simulink model "BaseEngineController_LS"  (Simulink 7.7)
settings: Solver=FixedStepDiscrete  StartTime=0.0  StopTime=10.0  RelTol=1e-3
PreLoadFcn:
  | try, eval([bdroot '_setup']); catch, eval('model_setup', ''); end
InitFcn:
  | try, eval([bdroot '_setup']); catch, eval('model_setup', ''); end
undefined symbols (not defined in the file): ECU555, High, motohawk_build_version, motohawk_trunc_name, motohawk_vardec_config_group, motohawk_vardec_path, True
libraries: MotoHawk_lib x1418, motohawk_control_primitives_lib x183, motohawk_engine_lib x32, simulink x21, motohawk_annotations_lib x9, AutoDoc_lib x8, simulink_extras x4, motohawk_ccp_examples_lib x1, motohawk_control_primitives_motoshare_lib x1
(part 8 of 27)

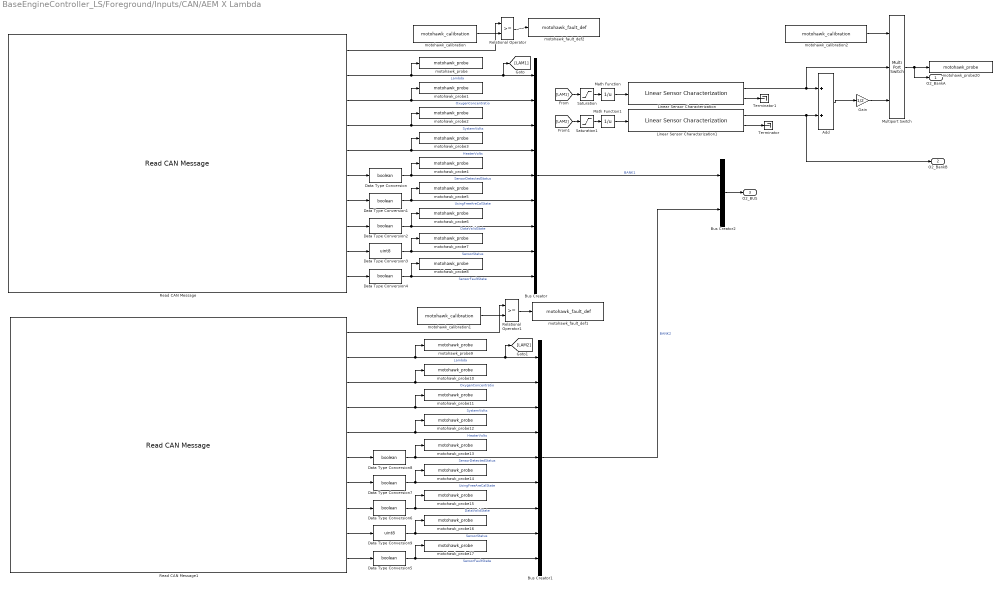
== system BaseEngineController_LS/Foreground/Inputs/CAN/AEM X Lambda ==
  Add : Sum
  Bus Creator : BusCreator  Inputs=9
  Bus Creator1 : BusCreator  Inputs=9
  Bus Creator2 : BusCreator  Inputs=2
  Data Type Conversion{,1..2,4..8} (8 alike) : DataTypeConversion  OutDataTypeStr=boolean
  Data Type Conversion3 : DataTypeConversion  OutDataTypeStr=uint8
  Data Type Conversion9 : DataTypeConversion  OutDataTypeStr=uint8
  Gain : Gain  Gain=1/2
  Linear Sensor Characterization : motohawk_engine_lib/Linear Sensor Characterization  SystemSampleTime=-1  nam='Bank1_EquivRatio'  prefix='Bank1_EquivRatio'  units='EquivRatio'  inputunits='EquivRatio'  parent_group=motohawk_vardec_path(gcb)  samp_time=-1
  Linear Sensor Characterization1 : motohawk_engine_lib/Linear Sensor Characterization  SystemSampleTime=-1  nam='Bank2_EquivRatio'  prefix='Bank2_EquivRatio'  units='EquivRatio'  inputunits='EquivRatio'  parent_group=motohawk_vardec_path(gcb)  samp_time=-1
  Math Function : Math  Operator=reciprocal  SaturateOnIntegerOverflow=on
  Math Function1 : Math  Operator=reciprocal  SaturateOnIntegerOverflow=on
  Multiport Switch : MultiPortSwitch  DataPortOrder=Zero-based contiguous  Inputs=2  zeroidx=on
  Read CAN Message : MotoHawk_lib/CAN Blocks/Read CAN Message  nam='CAN_1'  bus=-2  msg=CANRx_AEM_UEGO_1  queue=1  slot=''  valid=off  stale=on  labelwires=off
  Read CAN Message1 : MotoHawk_lib/CAN Blocks/Read CAN Message  nam='CAN_1'  bus=-2  msg=CANRx_AEM_UEGO_2  queue=1  slot=''  valid=off  stale=on  labelwires=off
  Relational Operator : RelationalOperator  OutDataTypeStr=boolean
  Relational Operator1 : RelationalOperator  OutDataTypeStr=boolean
  Saturation : Saturate  UpperLimit=inf  LowerLimit=.1
  Saturation1 : Saturate  UpperLimit=inf  LowerLimit=.1
  Terminator : Terminator
  Terminator1 : Terminator
  motohawk_calibration : MotoHawk_lib/Calibration & Probing Blocks/motohawk_calibration  nam='Lambda_1_Timeout'  val=100  storage=Calibration  show_more=on  name_source=Use Parameter  data_type=uint16  read_level=1  write_level=1  ovr_cals=on  view_as=Number  enum_struct={'Disabled', 'Enabled'}  vector_style=Wide Row  use_help_units=on  help=''  units='ms'  use_header_enum=off  row_header_enum={}  col_header_enum={}  use_min_max=off  min_val=-inf  max_val=inf  use_precision=off  precision=''  gain=1  offset=0  exp=1  use_mototune_group=off  mototune_group=motohawk_vardec_path(gcb)
  motohawk_calibration1 : MotoHawk_lib/Calibration & Probing Blocks/motohawk_calibration  nam='Lambda_2_Timeout'  val=100  storage=Calibration  show_more=on  name_source=Use Parameter  data_type=uint16  read_level=1  write_level=1  ovr_cals=on  view_as=Number  enum_struct={'Disabled', 'Enabled'}  vector_style=Wide Row  use_help_units=on  help=''  units='ms'  use_header_enum=off  row_header_enum={}  col_header_enum={}  use_min_max=off  min_val=-inf  max_val=inf  use_precision=off  precision=''  gain=1  offset=0  exp=1  use_mototune_group=off  mototune_group=motohawk_vardec_path(gcb)
  motohawk_calibration2 : MotoHawk_lib/Calibration & Probing Blocks/motohawk_calibration  nam='BankB_Avg_Enable'  val=1  storage=Calibration  show_more=on  name_source=Use Parameter  data_type=boolean  read_level=1  write_level=1  ovr_cals=on  view_as=Enumeration  enum_struct={'Disabled', 'Enabled'}  vector_style=Wide Row  use_help_units=off  help=''  units=''  use_header_enum=off  row_header_enum={}  col_header_enum={}  use_min_max=off  min_val=-inf  max_val=inf  use_precision=off  precision=''  gain=1  offset=0  exp=1  use_mototune_group=off  mototune_group=motohawk_vardec_path(gcb)
  motohawk_fault_def1 : MotoHawk_lib/Fault Management Blocks/motohawk_fault_def  nam='Lambda_2_Timeout'  mode=Enabled  id=[]  x=1  y=2  input_suspected=on  indeterminate=off  increment_xy=on  downsample_count=1  ovr_cals=on  ovr_actions=on  show_actions=on  action1_name=''  action1_cond=(None)  action2_name=''  action2_cond=(None)  action3_name=''  action3_cond=(None)  action4_name=''  action4_cond=(None)
  motohawk_fault_def2 : MotoHawk_lib/Fault Management Blocks/motohawk_fault_def  nam='Lambda_1_Timeout'  mode=Enabled  id=[]  x=1  y=2  input_suspected=on  indeterminate=off  increment_xy=on  downsample_count=1  ovr_cals=on  ovr_actions=on  show_actions=on  action1_name=''  action1_cond=(None)  action2_name=''  action2_cond=(None)  action3_name=''  action3_cond=(None)  action4_name=''  action4_cond=(None)
  motohawk_probe : MotoHawk_lib/Calibration & Probing Blocks/motohawk_probe  nam='Bank1_Lambda_Prb'  show_more=off  name_source=Use Parameter  read_level=1  view_as=Number  enum_struct={'Disabled', 'Enabled'}  vector_style=Wide Row  use_help_units=off  help=''  units=''  use_header_enum=off  row_header_enum={}  col_header_enum={}  use_precision=off  precision=''  gain=1  offset=0  exp=1  use_mototune_group=off  mototune_group=motohawk_vardec_path(gcb)
  motohawk_probe1 : MotoHawk_lib/Calibration & Probing Blocks/motohawk_probe  nam='Bank1_OxygenConcentration_Prb'  show_more=off  name_source=Use Parameter  read_level=1  view_as=Number  enum_struct={'Disabled', 'Enabled'}  vector_style=Wide Row  use_help_units=off  help=''  units=''  use_header_enum=off  row_header_enum={}  col_header_enum={}  use_precision=off  precision=''  gain=1  offset=0  exp=1  use_mototune_group=off  mototune_group=motohawk_vardec_path(gcb)
  motohawk_probe10 : MotoHawk_lib/Calibration & Probing Blocks/motohawk_probe  nam='Bank2_OxygenConcentration_Prb'  show_more=off  name_source=Use Parameter  read_level=1  view_as=Number  enum_struct={'Disabled', 'Enabled'}  vector_style=Wide Row  use_help_units=off  help=''  units=''  use_header_enum=off  row_header_enum={}  col_header_enum={}  use_precision=off  precision=''  gain=1  offset=0  exp=1  use_mototune_group=off  mototune_group=motohawk_vardec_path(gcb)
  motohawk_probe11 : MotoHawk_lib/Calibration & Probing Blocks/motohawk_probe  nam='Bank2_SystemVolts_Prb'  show_more=off  name_source=Use Parameter  read_level=1  view_as=Number  enum_struct={'Disabled', 'Enabled'}  vector_style=Wide Row  use_help_units=off  help=''  units=''  use_header_enum=off  row_header_enum={}  col_header_enum={}  use_precision=off  precision=''  gain=1  offset=0  exp=1  use_mototune_group=off  mototune_group=motohawk_vardec_path(gcb)
  motohawk_probe12 : MotoHawk_lib/Calibration & Probing Blocks/motohawk_probe  nam='Bank2_HeaterVolts_Prb'  show_more=off  name_source=Use Parameter  read_level=1  view_as=Number  enum_struct={'Disabled', 'Enabled'}  vector_style=Wide Row  use_help_units=off  help=''  units=''  use_header_enum=off  row_header_enum={}  col_header_enum={}  use_precision=off  precision=''  gain=1  offset=0  exp=1  use_mototune_group=off  mototune_group=motohawk_vardec_path(gcb)
  motohawk_probe13 : MotoHawk_lib/Calibration & Probing Blocks/motohawk_probe  nam='Bank2_SensorDetectedStatus_Prb'  show_more=off  name_source=Use Parameter  read_level=1  view_as=Number  enum_struct={'Disabled', 'Enabled'}  vector_style=Wide Row  use_help_units=off  help=''  units=''  use_header_enum=off  row_header_enum={}  col_header_enum={}  use_precision=off  precision=''  gain=1  offset=0  exp=1  use_mototune_group=off  mototune_group=motohawk_vardec_path(gcb)
  motohawk_probe14 : MotoHawk_lib/Calibration & Probing Blocks/motohawk_probe  nam='Bank2_UsingFreeAreCalState_Prb'  show_more=off  name_source=Use Parameter  read_level=1  view_as=Number  enum_struct={'Disabled', 'Enabled'}  vector_style=Wide Row  use_help_units=off  help=''  units=''  use_header_enum=off  row_header_enum={}  col_header_enum={}  use_precision=off  precision=''  gain=1  offset=0  exp=1  use_mototune_group=off  mototune_group=motohawk_vardec_path(gcb)
  motohawk_probe15 : MotoHawk_lib/Calibration & Probing Blocks/motohawk_probe  nam='Bank2_DataValidState_Prb'  show_more=off  name_source=Use Parameter  read_level=1  view_as=Number  enum_struct={'Disabled', 'Enabled'}  vector_style=Wide Row  use_help_units=off  help=''  units=''  use_header_enum=off  row_header_enum={}  col_header_enum={}  use_precision=off  precision=''  gain=1  offset=0  exp=1  use_mototune_group=off  mototune_group=motohawk_vardec_path(gcb)
  motohawk_probe16 : MotoHawk_lib/Calibration & Probing Blocks/motohawk_probe  nam='Bank2_SensorStatus_Prb'  show_more=on  name_source=Use Parameter  read_level=1  view_as=Enumeration  enum_struct={'Reset', 'WarmingUp', ' Stabilizing', 'ReadingNerstPumpImpedance', 'Equalizing', 'ReadingRcalValue', 'Run', 'Overheat', 'Overcool', 'HeaterShortCircuit', 'HeaterOpenCircuit', 'StartFreeAirCal', 'PerformingFreeAirCal', 'DetectingSensor', 'ReadingJunctionImpedance', 'EvapStartup', 'DeterminingSensorType', 'PreparingToRun','SaveSensor','NeedsNewFreeAirCal','Error'}  vector_style=Wide Row  use_help_units=off  help=''  units=''  use_header_enum=off  row_header_enum={}  col_header_enum={}  use_precision=off  precision=''  gain=1  offset=0  exp=1  use_mototune_group=off  mototune_group=motohawk_vardec_path(gcb)
  motohawk_probe17 : MotoHawk_lib/Calibration & Probing Blocks/motohawk_probe  nam='Bank2_SensorFaultState_Prb'  show_more=off  name_source=Use Parameter  read_level=1  view_as=Number  enum_struct={'Disabled', 'Enabled'}  vector_style=Wide Row  use_help_units=off  help=''  units=''  use_header_enum=off  row_header_enum={}  col_header_enum={}  use_precision=off  precision=''  gain=1  offset=0  exp=1  use_mototune_group=off  mototune_group=motohawk_vardec_path(gcb)
  motohawk_probe2 : MotoHawk_lib/Calibration & Probing Blocks/motohawk_probe  nam='Bank1_SystemVolts_Prb'  show_more=off  name_source=Use Parameter  read_level=1  view_as=Number  enum_struct={'Disabled', 'Enabled'}  vector_style=Wide Row  use_help_units=off  help=''  units=''  use_header_enum=off  row_header_enum={}  col_header_enum={}  use_precision=off  precision=''  gain=1  offset=0  exp=1  use_mototune_group=off  mototune_group=motohawk_vardec_path(gcb)
  motohawk_probe20 : MotoHawk_lib/Calibration & Probing Blocks/motohawk_probe  nam='O2_BankA_EquivRatio_Out'  show_more=off  name_source=Use Parameter  read_level=1  view_as=Number  enum_struct={'Disabled', 'Enabled'}  vector_style=Wide Row  use_help_units=off  help=''  units=''  use_header_enum=off  row_header_enum={}  col_header_enum={}  use_precision=off  precision=''  gain=1  offset=0  exp=1  use_mototune_group=off  mototune_group=motohawk_vardec_path(gcb)
  motohawk_probe3 : MotoHawk_lib/Calibration & Probing Blocks/motohawk_probe  nam='Bank1_HeaterVolts_Prb'  show_more=off  name_source=Use Parameter  read_level=1  view_as=Number  enum_struct={'Disabled', 'Enabled'}  vector_style=Wide Row  use_help_units=off  help=''  units=''  use_header_enum=off  row_header_enum={}  col_header_enum={}  use_precision=off  precision=''  gain=1  offset=0  exp=1  use_mototune_group=off  mototune_group=motohawk_vardec_path(gcb)
  motohawk_probe4 : MotoHawk_lib/Calibration & Probing Blocks/motohawk_probe  nam='Bank1_SensorDetectedStatus_Prb'  show_more=off  name_source=Use Parameter  read_level=1  view_as=Number  enum_struct={'Disabled', 'Enabled'}  vector_style=Wide Row  use_help_units=off  help=''  units=''  use_header_enum=off  row_header_enum={}  col_header_enum={}  use_precision=off  precision=''  gain=1  offset=0  exp=1  use_mototune_group=off  mototune_group=motohawk_vardec_path(gcb)
  motohawk_probe5 : MotoHawk_lib/Calibration & Probing Blocks/motohawk_probe  nam='Bank1_UsingFreeAreCalState_Prb'  show_more=off  name_source=Use Parameter  read_level=1  view_as=Number  enum_struct={'Disabled', 'Enabled'}  vector_style=Wide Row  use_help_units=off  help=''  units=''  use_header_enum=off  row_header_enum={}  col_header_enum={}  use_precision=off  precision=''  gain=1  offset=0  exp=1  use_mototune_group=off  mototune_group=motohawk_vardec_path(gcb)
  motohawk_probe6 : MotoHawk_lib/Calibration & Probing Blocks/motohawk_probe  nam='Bank1_DataValidState_Prb'  show_more=off  name_source=Use Parameter  read_level=1  view_as=Number  enum_struct={'Disabled', 'Enabled'}  vector_style=Wide Row  use_help_units=off  help=''  units=''  use_header_enum=off  row_header_enum={}  col_header_enum={}  use_precision=off  precision=''  gain=1  offset=0  exp=1  use_mototune_group=off  mototune_group=motohawk_vardec_path(gcb)
  motohawk_probe7 : MotoHawk_lib/Calibration & Probing Blocks/motohawk_probe  nam='Bank1_SensorStatus_Prb'  show_more=on  name_source=Use Parameter  read_level=1  view_as=Enumeration  enum_struct={'Reset', 'WarmingUp', ' Stabilizing', 'ReadingNerstPumpImpedance', 'Equalizing', 'ReadingRcalValue', 'Run', 'Overheat', 'Overcool', 'HeaterShortCircuit', 'HeaterOpenCircuit', 'StartFreeAirCal', 'PerformingFreeAirCal', 'DetectingSensor', 'ReadingJunctionImpedance', 'EvapStartup', 'DeterminingSensorType', 'PreparingToRun','SaveSensor','NeedsNewFreeAirCal','Error'}  vector_style=Wide Row  use_help_units=off  help=''  units=''  use_header_enum=off  row_header_enum={}  col_header_enum={}  use_precision=off  precision=''  gain=1  offset=0  exp=1  use_mototune_group=off  mototune_group=motohawk_vardec_path(gcb)
  motohawk_probe8 : MotoHawk_lib/Calibration & Probing Blocks/motohawk_probe  nam='Bank1_SensorFaultState_Prb'  show_more=off  name_source=Use Parameter  read_level=1  view_as=Number  enum_struct={'Disabled', 'Enabled'}  vector_style=Wide Row  use_help_units=off  help=''  units=''  use_header_enum=off  row_header_enum={}  col_header_enum={}  use_precision=off  precision=''  gain=1  offset=0  exp=1  use_mototune_group=off  mototune_group=motohawk_vardec_path(gcb)
  motohawk_probe9 : MotoHawk_lib/Calibration & Probing Blocks/motohawk_probe  nam='Bank2_Lambda_Prb'  show_more=off  name_source=Use Parameter  read_level=1  view_as=Number  enum_struct={'Disabled', 'Enabled'}  vector_style=Wide Row  use_help_units=off  help=''  units=''  use_header_enum=off  row_header_enum={}  col_header_enum={}  use_precision=off  precision=''  gain=1  offset=0  exp=1  use_mototune_group=off  mototune_group=motohawk_vardec_path(gcb)
  O2_BankA : Outport
  O2_BankB : Outport  Port=2
  O2_BUS : Outport  Port=3
  wires:
  Read CAN Message/1 -> Relational Operator/1
  motohawk_calibration/1 -> Relational Operator/2
  Relational Operator/1 -> motohawk_fault_def2/1
  Read CAN Message/2 -> motohawk_probe/1, Bus Creator/1, [LAM1]  "Lambda"
  Read CAN Message/3 -> motohawk_probe1/1, Bus Creator/2  "OxygenConcentratio"
  Read CAN Message/4 -> motohawk_probe2/1, Bus Creator/3  "SystemVolts"
  Read CAN Message/5 -> motohawk_probe3/1, Bus Creator/4  "HeaterVolts"
  Read CAN Message/6 -> Data Type Conversion/1
  Read CAN Message/7 -> Data Type Conversion1/1
  Read CAN Message/8 -> Data Type Conversion2/1
  Read CAN Message/9 -> Data Type Conversion3/1
  Read CAN Message/10 -> Data Type Conversion4/1
  Read CAN Message1/1 -> Relational Operator1/1
  motohawk_calibration1/1 -> Relational Operator1/2
  Relational Operator1/1 -> motohawk_fault_def1/1
  Read CAN Message1/2 -> motohawk_probe9/1, Bus Creator1/1, [LAM2]  "Lambda"
  Read CAN Message1/3 -> motohawk_probe10/1, Bus Creator1/2  "OxygenConcentratio"
  Read CAN Message1/4 -> motohawk_probe11/1, Bus Creator1/3  "SystemVolts"
  Read CAN Message1/5 -> motohawk_probe12/1, Bus Creator1/4  "HeaterVolts"
  Read CAN Message1/6 -> Data Type Conversion8/1
  Read CAN Message1/7 -> Data Type Conversion7/1
  Read CAN Message1/8 -> Data Type Conversion6/1
  Read CAN Message1/9 -> Data Type Conversion9/1
  Read CAN Message1/10 -> Data Type Conversion5/1
  Bus Creator/1 -> Bus Creator2/1  "BANK1"
  Bus Creator1/1 -> Bus Creator2/2  "BANK2"
  Bus Creator2/1 -> O2_BUS/1
  [LAM1] -> Saturation/1
  [LAM2] -> Saturation1/1
  Math Function/1 -> Linear Sensor Characterization/1
  Math Function1/1 -> Linear Sensor Characterization1/1
  Linear Sensor Characterization1/2 -> Terminator/1
  Linear Sensor Characterization/2 -> Terminator1/1
  Linear Sensor Characterization/1 -> Add/1, Multiport Switch/2
  Add/1 -> Gain/1
  motohawk_calibration2/1 -> Multiport Switch/1
  Saturation/1 -> Math Function/1
  Saturation1/1 -> Math Function1/1
  Linear Sensor Characterization1/1 -> Add/2, O2_BankB/1
  Multiport Switch/1 -> O2_BankA/1, motohawk_probe20/1
  Gain/1 -> Multiport Switch/3
  Data Type Conversion/1 -> motohawk_probe4/1, Bus Creator/5  "SensorDetectedStatus"
  Data Type Conversion1/1 -> motohawk_probe5/1, Bus Creator/6  "UsingFreeAreCalState"
  Data Type Conversion2/1 -> motohawk_probe6/1, Bus Creator/7  "DataValidState"
  Data Type Conversion3/1 -> motohawk_probe7/1, Bus Creator/8  "SensorStatus"
  Data Type Conversion4/1 -> motohawk_probe8/1, Bus Creator/9  "SensorFaultState"
  Data Type Conversion5/1 -> motohawk_probe17/1, Bus Creator1/9  "SensorFaultState"
  Data Type Conversion6/1 -> motohawk_probe15/1, Bus Creator1/7  "DataValidState"
  Data Type Conversion7/1 -> motohawk_probe14/1, Bus Creator1/6  "UsingFreeAreCalState"
  Data Type Conversion8/1 -> motohawk_probe13/1, Bus Creator1/5  "SensorDetectedStatus"
  Data Type Conversion9/1 -> motohawk_probe16/1, Bus Creator1/8  "SensorStatus"

== system BaseEngineController_LS/Foreground/Inputs/Digital/Scramble  ==
  ADC : Inport
  0 = No Inversion 1 = Inversion : MotoHawk_lib/Calibration & Probing Blocks/motohawk_calibration  nam=[prefix 'Polarity']  val=boolean(polarity-1)  storage=Calibration  show_more=on  name_source=Use Parameter  data_type=Inherit from 'Default Value'  read_level=1  write_level=1  ovr_cals=on  view_as=Number  enum_struct={'Disabled', 'Enabled'}  vector_style=Wide Row  use_help_units=on  help="'0 = High True    1 = Low True'"  units='bool'  use_header_enum=off  row_header_enum={}  col_header_enum={}  use_min_max=off  min_val=-inf  max_val=inf  use_precision=off  precision=''  gain=1  offset=0  exp=1  use_mototune_group=on  mototune_group=[group ' | ' nam ' Config']
  Button Delay 1 : Subsystem
  Data Type Conversion : DataTypeConversion  SaturateOnIntegerOverflow=on  RndMeth=Zero
  Logical Operator : Logic  Operator=XOR
  Override in Engineering Units : MotoHawk_lib/Calibration & Probing Blocks/motohawk_override_abs  SystemSampleTime=-1  parent_name=nam  parent_val=0  show_more=on  name_source=Use Parameter  parent_read_level=1  parent_override_level=1  view_as=Number  enum_struct={'Disabled', 'Enabled'}  use_help_units=on  parent_help='Override actuator, in engineering units'  parent_units='Boolean'  use_min_max=off  parent_min=-inf  parent_max=inf  use_precision=off  parent_precision=''  parent_gain=1  parent_offset=0  parent_exp=1  use_mototune_group=on  parent_group=group
  Relational Operator : RelationalOperator  Operator=>
  SwitchPoint : MotoHawk_lib/Calibration & Probing Blocks/motohawk_calibration  nam=[prefix 'SwitchPt']  val=switchpoint  storage=Calibration  show_more=on  name_source=Use Parameter  data_type=Inherit from 'Default Value'  read_level=1  write_level=1  ovr_cals=on  view_as=Number  enum_struct={'Disabled', 'Enabled'}  vector_style=Wide Row  use_help_units=on  help='Defines switch point in ADC units boolean conversion'  units='ADC'  use_header_enum=off  row_header_enum={}  col_header_enum={}  use_min_max=off  min_val=-inf  max_val=inf  use_precision=off  precision=''  gain=1  offset=0  exp=1  use_mototune_group=on  mototune_group=[group ' | ' nam ' Config']
  motohawk_calibration7 : MotoHawk_lib/Calibration & Probing Blocks/motohawk_calibration  nam='ScrambleDebounceDelay'  val=0.08  storage=Calibration  show_more=on  name_source=Use Parameter  data_type=Inherit from 'Default Value'  read_level=1  write_level=1  ovr_cals=on  view_as=Number  enum_struct={'Disabled', 'Enabled'}  vector_style=Wide Row  use_help_units=on  help='Cruise control debounce time'  units='S'  use_header_enum=off  row_header_enum={}  col_header_enum={}  use_min_max=off  min_val=-inf  max_val=inf  use_precision=off  precision=''  gain=1  offset=0  exp=1  use_mototune_group=off  mototune_group=motohawk_vardec_path(gcb)
  motohawk_probe : MotoHawk_lib/Calibration & Probing Blocks/motohawk_probe  nam=nam  show_more=on  name_source=Use Parameter  read_level=1  view_as=Number  enum_struct={'Disabled', 'Enabled'}  vector_style=Wide Row  use_help_units=on  help='Display output in engineering units'  units='Boolean'  use_header_enum=off  row_header_enum={}  col_header_enum={}  use_precision=off  precision=''  gain=1  offset=0  exp=1  use_mototune_group=on  mototune_group=group
  motohawk_probe1 : MotoHawk_lib/Calibration & Probing Blocks/motohawk_probe  nam=[nam '_Raw']  show_more=on  name_source=Use Parameter  read_level=1  view_as=Number  enum_struct={'Disabled', 'Enabled'}  vector_style=Wide Row  use_help_units=on  help='Display output in engineering units'  units='ADC'  use_header_enum=off  row_header_enum={}  col_header_enum={}  use_precision=off  precision=''  gain=1  offset=0  exp=1  use_mototune_group=on  mototune_group=group
  DiscOut : Outport
  wires:
  ADC/1 -> Data Type Conversion/1
  0 = No Inversion 1 = Inversion/1 -> Logical Operator/2
  Relational Operator/1 -> Logical Operator/1
  SwitchPoint/1 -> Relational Operator/2
  Override in Engineering Units/1 -> DiscOut/1, motohawk_probe/1
  Data Type Conversion/1 -> Relational Operator/1, motohawk_probe1/1
  motohawk_calibration7/1 -> Button Delay 1/2(Time)
  Logical Operator/1 -> Button Delay 1/1(In1)
  Button Delay 1/1(Out1) -> Override in Engineering Units/1

== system BaseEngineController_LS/Foreground/Inputs/Digital/VSPD_Filt ==
  In1 : Inport
  Abs : Abs
  Abs1 : Abs
  Abs2 : Abs
  Derivitive : motohawk_control_primitives_lib/Derivitive  SystemSampleTime=-1  samp_time=-1
  Logical Operator : Logic  AllPortsSameDT=off  OutDataTypeStr=boolean
  Logical Operator1 : Logic  Operator=OR  AllPortsSameDT=off  OutDataTypeStr=boolean
  Logical Operator2 : Logic  AllPortsSameDT=off  OutDataTypeStr=boolean
  Logical Operator3 : Logic  AllPortsSameDT=off  OutDataTypeStr=boolean
  Logical Operator5 : Logic  Operator=OR  AllPortsSameDT=off  OutDataTypeStr=boolean
  Relational Operator : RelationalOperator  OutDataTypeStr=boolean
  Relational Operator1 : RelationalOperator  Operator=<=  OutDataTypeStr=boolean
  Relational Operator2 : RelationalOperator  OutDataTypeStr=boolean
  Relational Operator3 : RelationalOperator  OutDataTypeStr=boolean
  S-R Flip-Flop : simulink_extras/Flip Flops/S-R Flip-Flop  SystemSampleTime=-1  initial_condition=0
  Sum : Sum  Inputs=+-
  Switch : Switch  Criteria=u2 ~= 0
  Terminator : Terminator
  Time Since Enabled (With Input)1 : motohawk_control_primitives_lib/Time Since Enabled (With Input)1  SystemSampleTime=-1  nam='TimeSinceVSPDReject'  samp_time=-1  init=0  upperlim=16000
  Unit Delay{,1..3} (4 alike) : UnitDelay  SampleTime=-1
  motohawk_calibration1 : MotoHawk_lib/Calibration & Probing Blocks/motohawk_calibration  nam='VSPD_RateReject_Enable'  val=1  storage=Calibration  show_more=on  name_source=Use Parameter  data_type=boolean  read_level=1  write_level=1  ovr_cals=on  view_as=Enumeration  enum_struct={'Disabled', 'Enabled'}  vector_style=Wide Row  use_help_units=on  help='Enable for if VSPD changes by more than this per/second ignore it'  units='enum'  use_header_enum=off  row_header_enum={}  col_header_enum={}  use_min_max=off  min_val=-inf  max_val=inf  use_precision=off  precision=''  gain=1  offset=0  exp=1  use_mototune_group=off  mototune_group=motohawk_vardec_path(gcb)
  motohawk_calibration2 : MotoHawk_lib/Calibration & Probing Blocks/motohawk_calibration  nam='VSPD_RateReject'  val=300  storage=Calibration  show_more=on  name_source=Use Parameter  data_type=Inherit via back propagation  read_level=1  write_level=1  ovr_cals=on  view_as=Number  enum_struct={'Disabled', 'Enabled'}  vector_style=Wide Row  use_help_units=on  help='If VSPD changes by more than this per/second ignore it'  units='mph/s'  use_header_enum=off  row_header_enum={}  col_header_enum={}  use_min_max=off  min_val=-inf  max_val=inf  use_precision=off  precision=''  gain=1  offset=0  exp=1  use_mototune_group=off  mototune_group=motohawk_vardec_path(gcb)
  motohawk_calibration3 : MotoHawk_lib/Calibration & Probing Blocks/motohawk_calibration  nam='VSPD_ZeroSpeed'  val=0.01  storage=Calibration  show_more=on  name_source=Use Parameter  data_type=Inherit from 'Default Value'  read_level=1  write_level=1  ovr_cals=on  view_as=Number  enum_struct={'Disabled', 'Enabled'}  vector_style=Wide Row  use_help_units=on  help='What VSPD filter considers zero speed'  units='mph'  use_header_enum=off  row_header_enum={}  col_header_enum={}  use_min_max=off  min_val=-inf  max_val=inf  use_precision=off  precision=''  gain=1  offset=0  exp=1  use_mototune_group=off  mototune_group=motohawk_vardec_path(gcb)
  motohawk_calibration4 : MotoHawk_lib/Calibration & Probing Blocks/motohawk_calibration  nam='VPSD_ChangeReject'  val=10  storage=Calibration  show_more=on  name_source=Use Parameter  data_type=Inherit via back propagation  read_level=1  write_level=1  ovr_cals=on  view_as=Number  enum_struct={'Disabled', 'Enabled'}  vector_style=Wide Row  use_help_units=on  help='If VSPD changes by more than this per/second ignore it'  units='mph/s'  use_header_enum=off  row_header_enum={}  col_header_enum={}  use_min_max=off  min_val=-inf  max_val=inf  use_precision=off  precision=''  gain=1  offset=0  exp=1  use_mototune_group=off  mototune_group=motohawk_vardec_path(gcb)
  motohawk_calibration5 : MotoHawk_lib/Calibration & Probing Blocks/motohawk_calibration  nam='VSPD_ChangeReject_Enable'  val=1  storage=Calibration  show_more=on  name_source=Use Parameter  data_type=boolean  read_level=1  write_level=1  ovr_cals=on  view_as=Enumeration  enum_struct={'Disabled', 'Enabled'}  vector_style=Wide Row  use_help_units=on  help='Enable for if VSPD changes by more than this per/second ignore it'  units='enum'  use_header_enum=off  row_header_enum={}  col_header_enum={}  use_min_max=off  min_val=-inf  max_val=inf  use_precision=off  precision=''  gain=1  offset=0  exp=1  use_mototune_group=off  mototune_group=motohawk_vardec_path(gcb)
  motohawk_calibration6 : MotoHawk_lib/Calibration & Probing Blocks/motohawk_calibration  nam='VSPD_RejectHoldTime'  val=1  storage=Calibration  show_more=on  name_source=Use Parameter  data_type=uint8  read_level=1  write_level=1  ovr_cals=on  view_as=Number  enum_struct={'Disabled', 'Enabled'}  vector_style=Wide Row  use_help_units=on  help='TimeToHoldLastValue'  units='sec'  use_header_enum=off  row_header_enum={}  col_header_enum={}  use_min_max=off  min_val=-inf  max_val=inf  use_precision=off  precision=''  gain=1  offset=0  exp=1  use_mototune_group=off  mototune_group=motohawk_vardec_path(gcb)
  motohawk_probe : MotoHawk_lib/Calibration & Probing Blocks/motohawk_probe  nam='VSPD_RateReject_Enabled'  show_more=off  name_source=Use Parameter  read_level=1  view_as=Number  enum_struct={'Disabled', 'Enabled'}  vector_style=Wide Row  use_help_units=off  help=''  units=''  use_header_enum=off  row_header_enum={}  col_header_enum={}  use_precision=off  precision=''  gain=1  offset=0  exp=1  use_mototune_group=off  mototune_group=motohawk_vardec_path(gcb)
  motohawk_probe1 : MotoHawk_lib/Calibration & Probing Blocks/motohawk_probe  nam='VSPD_ChangeReject_Enabled'  show_more=off  name_source=Use Parameter  read_level=1  view_as=Number  enum_struct={'Disabled', 'Enabled'}  vector_style=Wide Row  use_help_units=off  help=''  units=''  use_header_enum=off  row_header_enum={}  col_header_enum={}  use_precision=off  precision=''  gain=1  offset=0  exp=1  use_mototune_group=off  mototune_group=motohawk_vardec_path(gcb)
  motohawk_probe2 : MotoHawk_lib/Calibration & Probing Blocks/motohawk_probe  nam='VSPD_DigFinal'  show_more=off  name_source=Use Parameter  read_level=1  view_as=Number  enum_struct={'Disabled', 'Enabled'}  vector_style=Wide Row  use_help_units=off  help=''  units=''  use_header_enum=off  row_header_enum={}  col_header_enum={}  use_precision=off  precision=''  gain=1  offset=0  exp=1  use_mototune_group=off  mototune_group=motohawk_vardec_path(gcb)
  Out1 : Outport
  wires:
  In1/1 -> Derivitive/1, Sum/1, Abs1/1, Unit Delay1/1, Unit Delay3/1
  Derivitive/1 -> Abs/1
  Abs/1 -> Relational Operator/1
  motohawk_calibration2/1 -> Relational Operator/2
  Switch/1 -> Unit Delay/1, motohawk_probe2/1, Out1/1
  Unit Delay/1 -> Switch/1
  Relational Operator/1 -> Logical Operator/1
  motohawk_calibration1/1 -> Logical Operator/2
  Unit Delay1/1 -> Sum/2
  Abs1/1 -> Relational Operator1/1
  motohawk_calibration3/1 -> Relational Operator1/2
  Sum/1 -> Abs2/1
  motohawk_calibration4/1 -> Relational Operator2/2
  Abs2/1 -> Relational Operator2/1
  Relational Operator2/1 -> Logical Operator2/1
  Relational Operator1/1 -> Logical Operator2/2
  Logical Operator2/1 -> Logical Operator3/1
  motohawk_calibration5/1 -> Logical Operator3/2
  Logical Operator1/1 -> Logical Operator5/2, S-R Flip-Flop/1
  Logical Operator/1 -> Logical Operator1/1, motohawk_probe/1
  Logical Operator3/1 -> Logical Operator1/2, motohawk_probe1/1
  Time Since Enabled (With Input)1/1 -> Relational Operator3/1
  motohawk_calibration6/1 -> Relational Operator3/2
  S-R Flip-Flop/1 -> Logical Operator5/1, Time Since Enabled (With Input)1/1
  Logical Operator5/1 -> Switch/2
  Relational Operator3/1 -> Unit Delay2/1
  Unit Delay2/1 -> S-R Flip-Flop/2
  S-R Flip-Flop/2 -> Terminator/1
  Unit Delay3/1 -> Switch/3

== system BaseEngineController_LS/Foreground/Inputs/EngineSpeed/Encoder Diagnostics ==
  Encoder Fault : Inport
  CamEdges : motohawk_control_primitives_lib/CompareTo  SystemSampleTime=-1  op===  val=4
  CamSync : motohawk_control_primitives_lib/CompareTo  SystemSampleTime=-1  op===  val=5
  CounterThresh : motohawk_control_primitives_lib/CompareTo  SystemSampleTime=-1  op=>  val=100
  CrankEdges : motohawk_control_primitives_lib/CompareTo  SystemSampleTime=-1  op===  val=3
  CrankSync : motohawk_control_primitives_lib/CompareTo  SystemSampleTime=-1  op===  val=1
  Logical Operator{,1..3} (4 alike) : Logic  AllPortsSameDT=off  OutDataTypeStr=boolean
  motohawk_encoder_fault_trigger : MotoHawk_lib/Encoder Blocks/motohawk_encoder_fault_trigger  Tag=Trigger  inherited=on
  motohawk_fault_def : MotoHawk_lib/Fault Management Blocks/motohawk_fault_def  nam='CrankSyncFault'  mode=Enabled  id=[]  x=25  y=50  input_suspected=on  indeterminate=off  increment_xy=on  downsample_count=1  ovr_cals=on  ovr_actions=on  show_actions=off  action1_name=''  action1_cond=(None)  action2_name=''  action2_cond=(None)  action3_name=''  action3_cond=(None)  action4_name=''  action4_cond=(None)
  motohawk_fault_def1 : MotoHawk_lib/Fault Management Blocks/motohawk_fault_def  nam='CrankEdgesFault'  mode=Enabled  id=[]  x=25  y=50  input_suspected=on  indeterminate=off  increment_xy=on  downsample_count=1  ovr_cals=on  ovr_actions=on  show_actions=off  action1_name=''  action1_cond=(None)  action2_name=''  action2_cond=(None)  action3_name=''  action3_cond=(None)  action4_name=''  action4_cond=(None)
  motohawk_fault_def2 : MotoHawk_lib/Fault Management Blocks/motohawk_fault_def  nam='CamEdgesFault'  mode=Enabled  id=[]  x=25  y=50  input_suspected=on  indeterminate=off  increment_xy=on  downsample_count=1  ovr_cals=on  ovr_actions=on  show_actions=off  action1_name=''  action1_cond=(None)  action2_name=''  action2_cond=(None)  action3_name=''  action3_cond=(None)  action4_name=''  action4_cond=(None)
  motohawk_fault_def3 : MotoHawk_lib/Fault Management Blocks/motohawk_fault_def  nam='CamSyncFault'  mode=Enabled  id=[]  x=25  y=50  input_suspected=on  indeterminate=off  increment_xy=on  downsample_count=1  ovr_cals=on  ovr_actions=on  show_actions=off  action1_name=''  action1_cond=(None)  action2_name=''  action2_cond=(None)  action3_name=''  action3_cond=(None)  action4_name=''  action4_cond=(None)
  motohawk_model_probe_eval_f : Subsystem  AncestorBlock=MotoHawk_lib/Extra Development Blocks/motohawk_model_probe_eval_f  TreatAsAtomicUnit=on  mask(MotoHawk Debug Probe){nam='EncoderFaultCount', group=motohawk_vardec_path(gcb)}
      mask prompts: nam "Probe Name:"; group "MotoTune Group:"
      mask help:
      | Drops in a simple counter, visible from MotoTune, to see if the current subsystem is executing.
      |
      | The default expression for the Probe Name uses the name of the current subsystem (without spaces).
      |
      | ---------------------------------------------------------------------
      | Copyright 2005 MotoTron, Inc.  All Rights Reserved.
      mask init:
      | lbl = ['Debug Counter\nName: ' nam];
      mask Help: eval('motohawk_block_help(get_param(gcb,''MaskType''))');
      mask Display:
      | patch([0 0 1 1], [0 1 1 0], [220/255 220/255 220/255])
      | patch([0 0 1 1], [0 0.075 0.075 0], [230/255 0/255 0/255])
      | patch([0 0 1 1], [0.025 0.05 0.05 0.025], [150/255 0/255 0/255])
      | patch([0 0 1 1], [0 0.025 0.025 0], [0/255 0/255 0/255])
      | 
      | disp(lbl);
  motohawk_probe3 : MotoHawk_lib/Calibration & Probing Blocks/motohawk_probe  nam='EncoderFault'  show_more=on  name_source=Use Parameter  read_level=1  view_as=Enumeration  enum_struct={'No Fault','Crank Sync Fault','Reverse Rotation Fault','No Crank Edges Fault','No CAM edges fault','Cam Sync Fault'}  vector_style=Wide Row  use_help_units=off  help=''  units=''  use_header_enum=off  row_header_enum={}  col_header_enum={}  use_precision=off  precision=''  gain=1  offset=0  exp=1  use_mototune_group=on  mototune_group=motohawk_vardec_path(gcb)
  wires:
  Logical Operator3/1 -> motohawk_fault_def3/1
  CamSync/1 -> Logical Operator3/2
  Logical Operator2/1 -> motohawk_fault_def2/1
  CamEdges/1 -> Logical Operator2/2
  Logical Operator1/1 -> motohawk_fault_def1/1
  CrankEdges/1 -> Logical Operator1/2
  Encoder Fault/1 -> CamSync/1, CamEdges/1, CrankEdges/1, motohawk_probe3/1, CrankSync/1
  motohawk_encoder_fault_trigger/1 -> motohawk_model_probe_eval_f/Trigger
  motohawk_model_probe_eval_f/1(Count) -> CounterThresh/1
  Logical Operator/1 -> motohawk_fault_def/1
  CrankSync/1 -> Logical Operator/2
  CounterThresh/1 -> Logical Operator3/1, Logical Operator2/1, Logical Operator1/1, Logical Operator/1

== system BaseEngineController_LS/Foreground/Inputs/LinearSensors/FuelOxygenationSensor ==
  note: Linear Scaling from ADC Counts
      | to Engineering Units
  note: Faults for
      | Out-of-Range
      | Input
  ADC : Inport
  Data Type Conversion : DataTypeConversion  SaturateOnIntegerOverflow=on  RndMeth=Zero
  Filter Options : Subsystem
  Final Value : MotoHawk_lib/Calibration & Probing Blocks/motohawk_probe  nam=nam  show_more=on  name_source=Use Parameter  read_level=1  view_as=Number  enum_struct={'Disabled', 'Enabled'}  vector_style=Wide Row  use_help_units=on  help='Final value after Linear Sensor Characterization'  units=units  use_header_enum=off  row_header_enum={}  col_header_enum={}  use_precision=off  precision=''  gain=1  offset=0  exp=1  use_mototune_group=on  mototune_group=group
  From Analog Input : MotoHawk_lib/Calibration & Probing Blocks/motohawk_probe  nam=[prefix 'ADC']  show_more=on  name_source=Use Parameter  read_level=1  view_as=Number  enum_struct={'Disabled', 'Enabled'}  vector_style=Wide Row  use_help_units=on  help='Singal measured directly from sensor'  units=inputunits  use_header_enum=off  row_header_enum={}  col_header_enum={}  use_precision=off  precision=''  gain=1  offset=0  exp=1  use_mototune_group=on  mototune_group=group
  If : If  NumInputs=2  IfExpression=u1  ElseIfExpressions=u2  ZeroCross=off
  If Action Subsystem : Subsystem  TreatAsAtomicUnit=on
      mask Display: disp('Saturate');
  If Action Subsystem1 : Subsystem  TreatAsAtomicUnit=on
      mask Display: disp('Default');
  If Action Subsystem2 : Subsystem  TreatAsAtomicUnit=on
      mask Display: disp('Pass Through');
  Logical Operator1 : Logic  Operator=OR
  Logical Operator2 : Logic
  Logical Operator3 : Logic
  Logical Operator4 : Logic  Operator=OR
  Logical Operator5 : Logic
  Logical Operator6 : Logic  Operator=NOT
  Merge : Merge  Inputs=3
  Override : MotoHawk_lib/Calibration & Probing Blocks/motohawk_override_abs  SystemSampleTime=-1  parent_name=nam  parent_val=0  show_more=on  name_source=Use Parameter  parent_read_level=1  parent_override_level=1  view_as=Number  enum_struct={'Disabled', 'Enabled'}  use_help_units=on  parent_help='Override result of linear sensor characterization, in engineering units'  parent_units=units  use_min_max=on  parent_min=-inf  parent_max=inf  use_precision=off  parent_precision=''  parent_gain=1  parent_offset=0  parent_exp=1  use_mototune_group=on  parent_group=group
  Product1 : Product  SaturateOnIntegerOverflow=on  InputSameDT=on  OutDataTypeStr=Inherit: Same as first input
  Relational Operator2 : RelationalOperator  Operator=>  ZeroCross=off  InputSameDT=on
  Relational Operator3 : RelationalOperator  Operator=<  ZeroCross=off  InputSameDT=on
  Saturation : Saturate  UpperLimit=90  LowerLimit=0
  Sum1 : Sum  Inputs=|++  SaturateOnIntegerOverflow=on
  "Unfiltered, Before Range Checking" : MotoHawk_lib/Calibration & Probing Blocks/motohawk_probe  nam=[prefix 'Raw']  show_more=on  name_source=Use Parameter  read_level=1  view_as=Number  enum_struct={'Disabled', 'Enabled'}  vector_style=Wide Row  use_help_units=on  help='After conversion to engineering units, before range checking'  units=units  use_header_enum=off  row_header_enum={}  col_header_enum={}  use_precision=off  precision=''  gain=1  offset=0  exp=1  use_mototune_group=on  mototune_group=group
  Unit Delay1 : UnitDelay  SampleTime=-1
  motohawk_calibration1 : MotoHawk_lib/Calibration & Probing Blocks/motohawk_calibration  nam=[prefix 'InputHiFltPos']  val=1020  storage=Calibration  show_more=on  name_source=Use Parameter  data_type=double  read_level=1  write_level=1  ovr_cals=on  view_as=Number  enum_struct={'Disabled', 'Enabled'}  vector_style=Wide Row  use_help_units=on  help='Maximum allowable input, indicating short or open circuit'  units=inputunits  use_header_enum=off  row_header_enum={}  col_header_enum={}  use_min_max=off  min_val=-inf  max_val=inf  use_precision=off  precision=''  gain=1  offset=0  exp=1  use_mototune_group=on  mototune_group=[group ' | ' nam ' Config']
  motohawk_calibration3 : MotoHawk_lib/Calibration & Probing Blocks/motohawk_calibration  nam=[prefix 'DfltValue']  val=1  storage=Calibration  show_more=on  name_source=Use Parameter  data_type=double  read_level=1  write_level=1  ovr_cals=on  view_as=Number  enum_struct={'Disabled', 'Enabled'}  vector_style=Wide Row  use_help_units=on  help="'This is the initial default value should the sensor be in fault on key-up.  Otherwise the sensors outputs the last value prior to faulting'"  units=units  use_header_enum=off  row_header_enum={}  col_header_enum={}  use_min_max=off  min_val=-inf  max_val=inf  use_precision=off  precision=''  gain=1  offset=0  exp=1  use_mototune_group=on  mototune_group=[group ' | ' nam ' Config']
  motohawk_calibration4 : MotoHawk_lib/Calibration & Probing Blocks/motohawk_calibration  nam=[prefix 'Gain']  val=1  storage=Calibration  show_more=on  name_source=Use Parameter  data_type=double  read_level=1  write_level=1  ovr_cals=on  view_as=Number  enum_struct={'Disabled', 'Enabled'}  vector_style=Wide Row  use_help_units=on  help='Scaling from A/D counts to engineering units'  units=[units '/ADC']  use_header_enum=off  row_header_enum={}  col_header_enum={}  use_min_max=off  min_val=-inf  max_val=inf  use_precision=on  precision='5.4'  gain=1  offset=0  exp=1  use_mototune_group=on  mototune_group=[group ' | ' nam ' Config']
  motohawk_calibration5 : MotoHawk_lib/Calibration & Probing Blocks/motohawk_calibration  nam=[prefix 'Ofst']  val=0  storage=Calibration  show_more=on  name_source=Use Parameter  data_type=double  read_level=1  write_level=1  ovr_cals=on  view_as=Number  enum_struct={'Disabled', 'Enabled'}  vector_style=Wide Row  use_help_units=on  help='Offset after gain in engineering units'  units=units  use_header_enum=off  row_header_enum={}  col_header_enum={}  use_min_max=off  min_val=-inf  max_val=inf  use_precision=off  precision=''  gain=1  offset=0  exp=1  use_mototune_group=on  mototune_group=[group ' | ' nam ' Config']
  motohawk_calibration6 : MotoHawk_lib/Calibration & Probing Blocks/motohawk_calibration  nam=[prefix 'InputLoFltPos']  val=10  storage=Calibration  show_more=on  name_source=Use Parameter  data_type=double  read_level=1  write_level=1  ovr_cals=on  view_as=Number  enum_struct={'Disabled', 'Enabled'}  vector_style=Wide Row  use_help_units=on  help='Minimum allowable input, indicating short or open circuit'  units=inputunits  use_header_enum=off  row_header_enum={}  col_header_enum={}  use_min_max=off  min_val=-inf  max_val=inf  use_precision=off  precision=''  gain=1  offset=0  exp=1  use_mototune_group=on  mototune_group=[group ' | ' nam ' Config']
  motohawk_data_read1 : MotoHawk_lib/Data Storage Blocks/motohawk_data_read  source=Lookup By Name  structure=Scalar  operation=Read entire data structure at once  sz_vec=4  sz_row=2  sz_col=3  typ=boolean  nam='MPRD'  checkNull=on  struct_inst_name='Struct1'  struct_nam='MyStruct'
  motohawk_fault_def2 : MotoHawk_lib/Fault Management Blocks/motohawk_fault_def  nam=[prefix 'RangeHigh']  mode=Enabled  id=[]  x=25  y=50  input_suspected=on  indeterminate=off  increment_xy=on  downsample_count=1  ovr_cals=on  ovr_actions=on  show_actions=off  action1_name=''  action1_cond=(None)  action2_name=''  action2_cond=(None)  action3_name=''  action3_cond=(None)  action4_name=''  action4_cond=(None)
  motohawk_fault_def3 : MotoHawk_lib/Fault Management Blocks/motohawk_fault_def  nam=[prefix 'RangeLow']  mode=Enabled  id=[]  x=25  y=50  input_suspected=on  indeterminate=off  increment_xy=on  downsample_count=1  ovr_cals=on  ovr_actions=on  show_actions=off  action1_name=''  action1_cond=(None)  action2_name=''  action2_cond=(None)  action3_name=''  action3_cond=(None)  action4_name=''  action4_cond=(None)
  motohawk_fault_status1 : MotoHawk_lib/Fault Management Blocks/motohawk_fault_status  source=Lookup By Name  nam=[prefix 'RangeHigh']  status=Active
  motohawk_fault_status2 : MotoHawk_lib/Fault Management Blocks/motohawk_fault_status  source=Lookup By Name  nam=[prefix 'RangeHigh']  status=Suspected
  motohawk_fault_status3 : MotoHawk_lib/Fault Management Blocks/motohawk_fault_status  source=Lookup By Name  nam=[prefix 'RangeLow']  status=Suspected
  motohawk_fault_status4 : MotoHawk_lib/Fault Management Blocks/motohawk_fault_status  source=Lookup By Name  nam=[prefix 'RangeLow']  status=Active
  EngUnitsFilt : Outport
  EngUnitsRaw : Outport  Port=2
  wires:
  Logical Operator4/1 -> If/2, Logical Operator6/1
  Logical Operator1/1 -> Logical Operator5/2
  Logical Operator5/1 -> If/1
  Logical Operator6/1 -> Logical Operator5/1
  Filter Options/1(Out1) -> Override/1
  motohawk_calibration3/1 -> If Action Subsystem1/1(In)
  Unit Delay1/1 -> If Action Subsystem/1(In)
  If/2 -> If Action Subsystem1/Action
  If Action Subsystem1/1(Out) -> Merge/3
  motohawk_fault_status4/1 -> Logical Operator4/2
  motohawk_fault_status1/1 -> Logical Operator4/1
  Sum1/1 -> "Unfiltered, Before Range Checking"/1, Saturation/1
  If Action Subsystem/1(Out) -> Merge/2
  If Action Subsystem2/1(Out) -> Merge/1
  motohawk_fault_status3/1 -> Logical Operator1/2
  motohawk_fault_status2/1 -> Logical Operator1/1
  motohawk_calibration6/1 -> Relational Operator3/2
  motohawk_calibration1/1 -> Relational Operator2/2
  Relational Operator2/1 -> Logical Operator2/2
  Relational Operator3/1 -> Logical Operator3/2
  Logical Operator2/1 -> motohawk_fault_def2/1
  Logical Operator3/1 -> motohawk_fault_def3/1
  motohawk_data_read1/1 -> Logical Operator3/1, Logical Operator2/1
  Product1/1 -> Sum1/1
  motohawk_calibration5/1 -> Sum1/2
  motohawk_calibration4/1 -> Product1/2
  Override/1 -> EngUnitsFilt/1, Final Value/1
  ADC/1 -> Data Type Conversion/1, From Analog Input/1
  Data Type Conversion/1 -> Product1/1, Relational Operator3/1, Relational Operator2/1
  If/1 -> If Action Subsystem/Action
  If/3 -> If Action Subsystem2/Action
  Merge/1 -> EngUnitsRaw/1, Unit Delay1/1, Filter Options/1(In1)
  Saturation/1 -> If Action Subsystem2/1(In)

== system BaseEngineController_LS/Foreground/Inputs/LinearSensors/MAP_Crank_Synchronous ==
  MID_TDC : Subsystem  TreatAsAtomicUnit=on
  Merge : Merge
  Once at Startup : Subsystem  TreatAsAtomicUnit=on
  motohawk_trigger2 : MotoHawk_lib/Trigger Blocks/motohawk_trigger  Tag=Trigger  trigger=STARTUP_EVENT  function_name=Trigger_STARTUP_EVENT_4486p0011  priority_order=0  inherited=on  run_disabled=off  override_app_monitor=off  target=ECU555_80
  motohawk_trigger5 : MotoHawk_lib/Trigger Blocks/motohawk_trigger  Tag=Trigger  trigger=FGND_MID_TDC_EVENT  function_name=Trigger_FGND_MID_TDC_EVENT_4487p0011  priority_order=0  inherited=on  run_disabled=off  override_app_monitor=off  target=ECU555_80
  ADC : Outport
  wires:
  motohawk_trigger5/1 -> MID_TDC/Trigger
  MID_TDC/1(ADC) -> Merge/2
  motohawk_trigger2/1 -> Once at Startup/Trigger
  Merge/1 -> ADC/1
  Once at Startup/1(ADC) -> Merge/1

== system BaseEngineController_LS/Foreground/Inputs/NonLinearSensors/Fuel Level ==
  function : TriggerPort  TriggerType=function-call
  "Fuel_Lvl  " : motohawk_engine_lib/Non-Linear Sensor Characterization (tbl)  SystemSampleTime=-1  nam='Fuel_Lvl'  prefix='Fuel_Lvl'  units='%'  inputunits='ADC'  parent_group=motohawk_vardec_path(gcb)  tblsize=5  samp_time=-1
  motohawk_ain : MotoHawk_lib/Analog I//O Blocks/motohawk_ain  res_name=[]  text_resource=AN15M  code_resource=RES_ECUP  val_resource=-1  target=ECU555-80  resource_enum_str=(None)=-1,ECUP=53,DRVP=54,XDRP=55,AN1M=56,AN2M=57,AN3M=58,AN4M=59,AN5M=60,AN6M=61,AN7M=62,AN8M=63,AN9M=64,AN10M=65,AN11M=66,AN12M=67,AN13M=68,AN14M=69,AN15M=70,AN16M=71,AN17M=72,AN18M=73,AN19M=74,O2A=90,O2B=91,XDRP_B=92  altref=5V Reference  typ=uint16  num_adc_bits=10  use_stat=off  use_vardec=on  nam='FuelLvlSensorPin'  read_level=1  write_level=1  group='System | I/O Pins | Inputs Config'
  Fuel Lvl : Outport
  Fuel Lvl Raw : Outport  Port=2
  wires:
  motohawk_ain/1 -> "Fuel_Lvl  "/1
  "Fuel_Lvl  "/1 -> Fuel Lvl/1
  "Fuel_Lvl  "/2 -> Fuel Lvl Raw/1
